simulink subsystem "ALU_64bit_v2_SS"  (R2022a)
settings: Solver=VariableStepAuto  StartTime=0.0  StopTime=10.0  RelTol=1e-3
libraries: hdlBasic x192
(part 1 of 3)
settings Model: Creator=viktor  LastModifiedBy=viktor

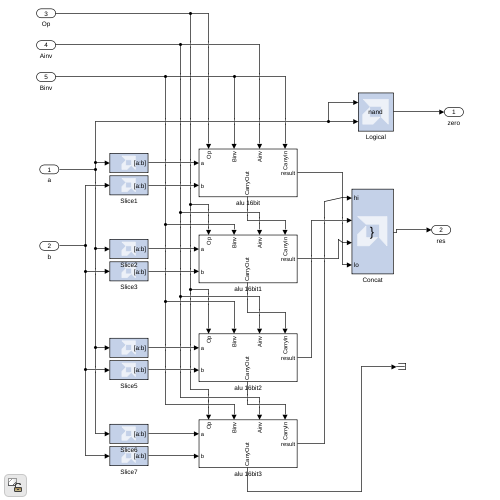
[thumbnail: Simulink's stored preview of the top-level diagram]
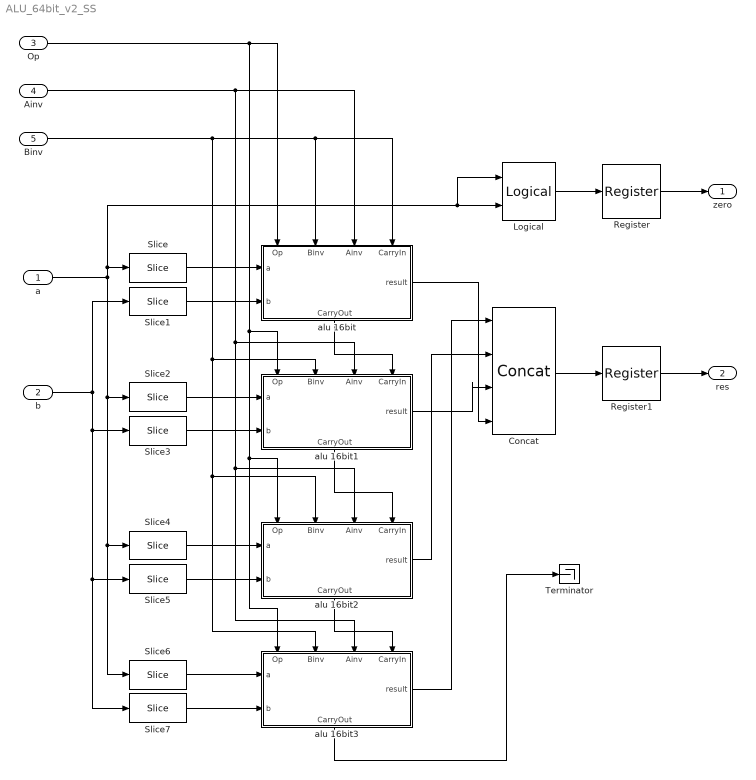
== system ALU_64bit_v2_SS ==
  a : Inport
  b : Inport  Port=2
  Op : Inport  Port=3
  Ainv : Inport  Port=4
  Binv : Inport  Port=5
  Concat : hdlBasic/Concat  num_inputs=4  XmcBlockStatus=1  maskContainerNames=group1  block_type=concat  block_config=sysgen:Concat_config
  Logical : hdlBasic/Logical  logical_function=NAND  inputs=2  en=off  latency=0  precision=User Defined  arith_type=Boolean  n_bits=16  bin_pt=0  align_bp=on  overflow=[]  quantization=[]  XmcBlockStatus=1  maskContainerNames=tabcontainer1  block_type=logical  block_config=sysgen:Logical_config
  Register : hdlBasic/Register  init=0  rst=off  en=off  XmcBlockStatus=1  maskContainerNames=tabcontainer1  block_type=register  block_config=sysgen:Register_config
  Register1 : hdlBasic/Register  init=0  rst=off  en=off  XmcBlockStatus=1  maskContainerNames=tabcontainer1  block_type=register  block_config=sysgen:Register_config
  Slice : hdlBasic/Slice  nbits=1  boolean_output=off  mode=Two Bit Locations  bit1=15  base1=LSB of Input  bit0=0  base0=LSB of Input  XmcBlockStatus=1  maskContainerNames=group1  block_type=slice  block_config=sysgen:Slice_config
  Slice1 : hdlBasic/Slice  nbits=1  boolean_output=off  mode=Two Bit Locations  bit1=15  base1=LSB of Input  bit0=0  base0=LSB of Input  XmcBlockStatus=1  maskContainerNames=group1  block_type=slice  block_config=sysgen:Slice_config
  Slice2 : hdlBasic/Slice  nbits=1  boolean_output=off  mode=Two Bit Locations  bit1=31  base1=LSB of Input  bit0=16  base0=LSB of Input  XmcBlockStatus=1  maskContainerNames=group1  block_type=slice  block_config=sysgen:Slice_config
  Slice3 : hdlBasic/Slice  nbits=1  boolean_output=off  mode=Two Bit Locations  bit1=31  base1=LSB of Input  bit0=16  base0=LSB of Input  XmcBlockStatus=1  maskContainerNames=group1  block_type=slice  block_config=sysgen:Slice_config
  Slice4 : hdlBasic/Slice  nbits=1  boolean_output=off  mode=Two Bit Locations  bit1=47  base1=LSB of Input  bit0=32  base0=LSB of Input  XmcBlockStatus=1  maskContainerNames=group1  block_type=slice  block_config=sysgen:Slice_config
  Slice5 : hdlBasic/Slice  nbits=1  boolean_output=off  mode=Two Bit Locations  bit1=47  base1=LSB of Input  bit0=32  base0=LSB of Input  XmcBlockStatus=1  maskContainerNames=group1  block_type=slice  block_config=sysgen:Slice_config
  Slice6 : hdlBasic/Slice  nbits=1  boolean_output=off  mode=Two Bit Locations  bit1=63  base1=LSB of Input  bit0=48  base0=LSB of Input  XmcBlockStatus=1  maskContainerNames=group1  block_type=slice  block_config=sysgen:Slice_config
  Slice7 : hdlBasic/Slice  nbits=1  boolean_output=off  mode=Two Bit Locations  bit1=63  base1=LSB of Input  bit0=48  base0=LSB of Input  XmcBlockStatus=1  maskContainerNames=group1  block_type=slice  block_config=sysgen:Slice_config
  Terminator : Terminator
  alu 16bit : Subsystem
      settings: PortSchema="{\"entries\":[{\"content\":{\"sides\":[{\"content\":{\"connectorIds\":[\"In1\",\"In2\"]},\"type\":\"ConnectorPlacement.EquallySpacedRectSide\",\"uuid\":\"2d8c2f3b-1550-46fa-bff2-1c6af3b5a107\"},{\"content\":{\"connectorIds\":[\"Out1\"],\"side\":\"RIGHT\"},\"type\":\"ConnectorPlacement.EquallySpacedRectSide\",\"uuid\":\"4b8f41aa-218a-4e29-bd3a-77a8547f4b37\"},{\"content\":{\"connectorIds\":[\"In3\",\"In4\",\"In5\",\"In6\"],\"side\":\"TOP\"},\"type\":\"ConnectorPlacement.EquallySpacedRectSide\",\"uuid\":\"e119eb8d-dd79-436a-880b-8e6ed91d7b6a\"},{\"content\":{\"connectorIds\":[\"Out2\"],\"side\":\"BOTTOM\"},\"type\":\"ConnectorPlacement.EquallySpacedRectSide\",\"uuid\":\"719cfc2d-1a88-4ba6-b6fd-9ae312fb718e\"}]},\"type\":\"ConnectorPlacement.EquallySpacedConnector\",\"uuid\":\"6756e4eb-c638-4708-925d-61f35342c635\"}],\"packageUris\":[\"http://schema.mathworks.com/mf0/Connector/R2020b\"],\"version\":\"1.0\"}"
  alu 16bit1 : Subsystem
      settings: PortSchema="{\"entries\":[{\"content\":{\"sides\":[{\"content\":{\"connectorIds\":[\"In1\",\"In2\"]},\"type\":\"ConnectorPlacement.EquallySpacedRectSide\",\"uuid\":\"2d8c2f3b-1550-46fa-bff2-1c6af3b5a107\"},{\"content\":{\"connectorIds\":[\"Out1\"],\"side\":\"RIGHT\"},\"type\":\"ConnectorPlacement.EquallySpacedRectSide\",\"uuid\":\"4b8f41aa-218a-4e29-bd3a-77a8547f4b37\"},{\"content\":{\"connectorIds\":[\"In3\",\"In4\",\"In5\",\"In6\"],\"side\":\"TOP\"},\"type\":\"ConnectorPlacement.EquallySpacedRectSide\",\"uuid\":\"e119eb8d-dd79-436a-880b-8e6ed91d7b6a\"},{\"content\":{\"connectorIds\":[\"Out2\"],\"side\":\"BOTTOM\"},\"type\":\"ConnectorPlacement.EquallySpacedRectSide\",\"uuid\":\"719cfc2d-1a88-4ba6-b6fd-9ae312fb718e\"}]},\"type\":\"ConnectorPlacement.EquallySpacedConnector\",\"uuid\":\"6756e4eb-c638-4708-925d-61f35342c635\"}],\"packageUris\":[\"http://schema.mathworks.com/mf0/Connector/R2020b\"],\"version\":\"1.0\"}"
  alu 16bit2 : Subsystem
      settings: PortSchema="{\"entries\":[{\"content\":{\"sides\":[{\"content\":{\"connectorIds\":[\"In1\",\"In2\"]},\"type\":\"ConnectorPlacement.EquallySpacedRectSide\",\"uuid\":\"2d8c2f3b-1550-46fa-bff2-1c6af3b5a107\"},{\"content\":{\"connectorIds\":[\"Out1\"],\"side\":\"RIGHT\"},\"type\":\"ConnectorPlacement.EquallySpacedRectSide\",\"uuid\":\"4b8f41aa-218a-4e29-bd3a-77a8547f4b37\"},{\"content\":{\"connectorIds\":[\"In3\",\"In4\",\"In5\",\"In6\"],\"side\":\"TOP\"},\"type\":\"ConnectorPlacement.EquallySpacedRectSide\",\"uuid\":\"e119eb8d-dd79-436a-880b-8e6ed91d7b6a\"},{\"content\":{\"connectorIds\":[\"Out2\"],\"side\":\"BOTTOM\"},\"type\":\"ConnectorPlacement.EquallySpacedRectSide\",\"uuid\":\"719cfc2d-1a88-4ba6-b6fd-9ae312fb718e\"}]},\"type\":\"ConnectorPlacement.EquallySpacedConnector\",\"uuid\":\"6756e4eb-c638-4708-925d-61f35342c635\"}],\"packageUris\":[\"http://schema.mathworks.com/mf0/Connector/R2020b\"],\"version\":\"1.0\"}"
  alu 16bit3 : Subsystem
      settings: PortSchema="{\"entries\":[{\"content\":{\"sides\":[{\"content\":{\"connectorIds\":[\"In1\",\"In2\"]},\"type\":\"ConnectorPlacement.EquallySpacedRectSide\",\"uuid\":\"2d8c2f3b-1550-46fa-bff2-1c6af3b5a107\"},{\"content\":{\"connectorIds\":[\"Out1\"],\"side\":\"RIGHT\"},\"type\":\"ConnectorPlacement.EquallySpacedRectSide\",\"uuid\":\"4b8f41aa-218a-4e29-bd3a-77a8547f4b37\"},{\"content\":{\"connectorIds\":[\"In3\",\"In4\",\"In5\",\"In6\"],\"side\":\"TOP\"},\"type\":\"ConnectorPlacement.EquallySpacedRectSide\",\"uuid\":\"e119eb8d-dd79-436a-880b-8e6ed91d7b6a\"},{\"content\":{\"connectorIds\":[\"Out2\"],\"side\":\"BOTTOM\"},\"type\":\"ConnectorPlacement.EquallySpacedRectSide\",\"uuid\":\"719cfc2d-1a88-4ba6-b6fd-9ae312fb718e\"}]},\"type\":\"ConnectorPlacement.EquallySpacedConnector\",\"uuid\":\"6756e4eb-c638-4708-925d-61f35342c635\"}],\"packageUris\":[\"http://schema.mathworks.com/mf0/Connector/R2020b\"],\"version\":\"1.0\"}"
  zero : Outport
  res : Outport  Port=2
  wires:
  Slice4/1 -> alu 16bit2/1(a)
  alu 16bit1/2(CarryOut) -> alu 16bit2/6(CarryIn)
  Slice1/1 -> alu 16bit/2(b)
  Slice6/1 -> alu 16bit3/1(a)
  alu 16bit3/2(CarryOut) -> Terminator/1
  Slice/1 -> alu 16bit/1(a)
  alu 16bit2/1(result) -> Concat/2
  Slice5/1 -> alu 16bit2/2(b)
  b/1 -> Slice1/1, Slice3/1, Slice5/1, Slice7/1
  Slice7/1 -> alu 16bit3/2(b)
  Slice2/1 -> alu 16bit1/1(a)
  alu 16bit2/2(CarryOut) -> alu 16bit3/6(CarryIn)
  Ainv/1 -> alu 16bit/5(Ainv), alu 16bit1/5(Ainv), alu 16bit2/5(Ainv), alu 16bit3/5(Ainv)
  a/1 -> Logical/1, Logical/2, Slice/1, Slice2/1, Slice4/1, Slice6/1
  alu 16bit1/1(result) -> Concat/3
  Slice3/1 -> alu 16bit1/2(b)
  alu 16bit/2(CarryOut) -> alu 16bit1/6(CarryIn)
  Op/1 -> alu 16bit/3(Op), alu 16bit1/3(Op), alu 16bit2/3(Op), alu 16bit3/3(Op)
  Logical/1 -> Register/1
  Binv/1 -> alu 16bit/6(CarryIn), alu 16bit/4(Binv), alu 16bit1/4(Binv), alu 16bit2/4(Binv), alu 16bit3/4(Binv)
  alu 16bit/1(result) -> Concat/4
  alu 16bit3/1(result) -> Concat/1
  Register/1 -> zero/1
  Concat/1 -> Register1/1
  Register1/1 -> res/1

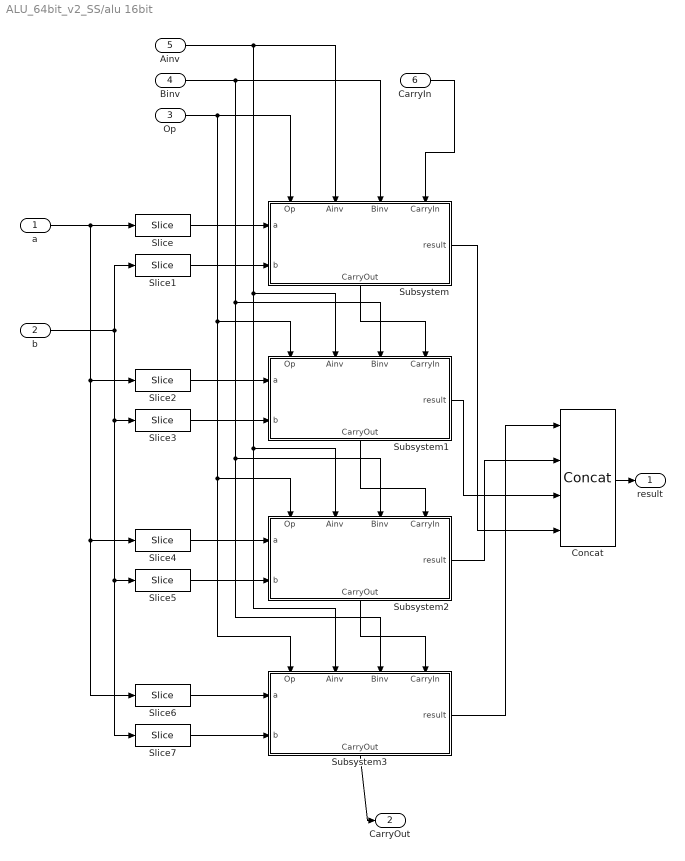
== system ALU_64bit_v2_SS/alu 16bit ==
  a : Inport
  b : Inport  Port=2
  Op : Inport  Port=3
  Binv : Inport  Port=4
  Ainv : Inport  Port=5
  CarryIn : Inport  Port=6
  Concat : hdlBasic/Concat  num_inputs=4  XmcBlockStatus=1  maskContainerNames=group1  block_type=concat  block_config=sysgen:Concat_config
  Slice : hdlBasic/Slice  nbits=1  boolean_output=off  mode=Two Bit Locations  bit1=3  base1=LSB of Input  bit0=0  base0=LSB of Input  XmcBlockStatus=1  maskContainerNames=group1  block_type=slice  block_config=sysgen:Slice_config
  Slice1 : hdlBasic/Slice  nbits=1  boolean_output=off  mode=Two Bit Locations  bit1=3  base1=LSB of Input  bit0=0  base0=LSB of Input  XmcBlockStatus=1  maskContainerNames=group1  block_type=slice  block_config=sysgen:Slice_config
  Slice2 : hdlBasic/Slice  nbits=1  boolean_output=off  mode=Two Bit Locations  bit1=7  base1=LSB of Input  bit0=4  base0=LSB of Input  XmcBlockStatus=1  maskContainerNames=group1  block_type=slice  block_config=sysgen:Slice_config
  Slice3 : hdlBasic/Slice  nbits=1  boolean_output=off  mode=Two Bit Locations  bit1=7  base1=LSB of Input  bit0=4  base0=LSB of Input  XmcBlockStatus=1  maskContainerNames=group1  block_type=slice  block_config=sysgen:Slice_config
  Slice4 : hdlBasic/Slice  nbits=1  boolean_output=off  mode=Two Bit Locations  bit1=11  base1=LSB of Input  bit0=8  base0=LSB of Input  XmcBlockStatus=1  maskContainerNames=group1  block_type=slice  block_config=sysgen:Slice_config
  Slice5 : hdlBasic/Slice  nbits=1  boolean_output=off  mode=Two Bit Locations  bit1=11  base1=LSB of Input  bit0=8  base0=LSB of Input  XmcBlockStatus=1  maskContainerNames=group1  block_type=slice  block_config=sysgen:Slice_config
  Slice6 : hdlBasic/Slice  nbits=1  boolean_output=off  mode=Two Bit Locations  bit1=15  base1=LSB of Input  bit0=12  base0=LSB of Input  XmcBlockStatus=1  maskContainerNames=group1  block_type=slice  block_config=sysgen:Slice_config
  Slice7 : hdlBasic/Slice  nbits=1  boolean_output=off  mode=Two Bit Locations  bit1=15  base1=LSB of Input  bit0=12  base0=LSB of Input  XmcBlockStatus=1  maskContainerNames=group1  block_type=slice  block_config=sysgen:Slice_config
  Subsystem : Subsystem
      settings: PortSchema="{\"entries\":[{\"content\":{\"sides\":[{\"content\":{\"connectorIds\":[\"In1\",\"In2\"]},\"type\":\"ConnectorPlacement.EquallySpacedRectSide\",\"uuid\":\"2d8c2f3b-1550-46fa-bff2-1c6af3b5a107\"},{\"content\":{\"connectorIds\":[\"Out1\"],\"side\":\"RIGHT\"},\"type\":\"ConnectorPlacement.EquallySpacedRectSide\",\"uuid\":\"4b8f41aa-218a-4e29-bd3a-77a8547f4b37\"},{\"content\":{\"connectorIds\":[\"In3\",\"In4\",\"In5\",\"In6\"],\"side\":\"TOP\"},\"type\":\"ConnectorPlacement.EquallySpacedRectSide\",\"uuid\":\"e119eb8d-dd79-436a-880b-8e6ed91d7b6a\"},{\"content\":{\"connectorIds\":[\"Out2\"],\"side\":\"BOTTOM\"},\"type\":\"ConnectorPlacement.EquallySpacedRectSide\",\"uuid\":\"1d45baa7-6d44-42d8-8289-fca13db264c9\"}]},\"type\":\"ConnectorPlacement.EquallySpacedConnector\",\"uuid\":\"6756e4eb-c638-4708-925d-61f35342c635\"}],\"packageUris\":[\"http://schema.mathworks.com/mf0/Connector/R2020b\"],\"version\":\"1.0\"}"
  Subsystem1 : Subsystem
      settings: PortSchema="{\"entries\":[{\"content\":{\"sides\":[{\"content\":{\"connectorIds\":[\"In1\",\"In2\"]},\"type\":\"ConnectorPlacement.EquallySpacedRectSide\",\"uuid\":\"2d8c2f3b-1550-46fa-bff2-1c6af3b5a107\"},{\"content\":{\"connectorIds\":[\"Out1\"],\"side\":\"RIGHT\"},\"type\":\"ConnectorPlacement.EquallySpacedRectSide\",\"uuid\":\"4b8f41aa-218a-4e29-bd3a-77a8547f4b37\"},{\"content\":{\"connectorIds\":[\"In3\",\"In4\",\"In5\",\"In6\"],\"side\":\"TOP\"},\"type\":\"ConnectorPlacement.EquallySpacedRectSide\",\"uuid\":\"e119eb8d-dd79-436a-880b-8e6ed91d7b6a\"},{\"content\":{\"connectorIds\":[\"Out2\"],\"side\":\"BOTTOM\"},\"type\":\"ConnectorPlacement.EquallySpacedRectSide\",\"uuid\":\"1d45baa7-6d44-42d8-8289-fca13db264c9\"}]},\"type\":\"ConnectorPlacement.EquallySpacedConnector\",\"uuid\":\"6756e4eb-c638-4708-925d-61f35342c635\"}],\"packageUris\":[\"http://schema.mathworks.com/mf0/Connector/R2020b\"],\"version\":\"1.0\"}"
  Subsystem2 : Subsystem
      settings: PortSchema="{\"entries\":[{\"content\":{\"sides\":[{\"content\":{\"connectorIds\":[\"In1\",\"In2\"]},\"type\":\"ConnectorPlacement.EquallySpacedRectSide\",\"uuid\":\"2d8c2f3b-1550-46fa-bff2-1c6af3b5a107\"},{\"content\":{\"connectorIds\":[\"Out1\"],\"side\":\"RIGHT\"},\"type\":\"ConnectorPlacement.EquallySpacedRectSide\",\"uuid\":\"4b8f41aa-218a-4e29-bd3a-77a8547f4b37\"},{\"content\":{\"connectorIds\":[\"In3\",\"In4\",\"In5\",\"In6\"],\"side\":\"TOP\"},\"type\":\"ConnectorPlacement.EquallySpacedRectSide\",\"uuid\":\"e119eb8d-dd79-436a-880b-8e6ed91d7b6a\"},{\"content\":{\"connectorIds\":[\"Out2\"],\"side\":\"BOTTOM\"},\"type\":\"ConnectorPlacement.EquallySpacedRectSide\",\"uuid\":\"1d45baa7-6d44-42d8-8289-fca13db264c9\"}]},\"type\":\"ConnectorPlacement.EquallySpacedConnector\",\"uuid\":\"6756e4eb-c638-4708-925d-61f35342c635\"}],\"packageUris\":[\"http://schema.mathworks.com/mf0/Connector/R2020b\"],\"version\":\"1.0\"}"
  Subsystem3 : Subsystem
      settings: PortSchema="{\"entries\":[{\"content\":{\"sides\":[{\"content\":{\"connectorIds\":[\"In1\",\"In2\"]},\"type\":\"ConnectorPlacement.EquallySpacedRectSide\",\"uuid\":\"2d8c2f3b-1550-46fa-bff2-1c6af3b5a107\"},{\"content\":{\"connectorIds\":[\"Out1\"],\"side\":\"RIGHT\"},\"type\":\"ConnectorPlacement.EquallySpacedRectSide\",\"uuid\":\"4b8f41aa-218a-4e29-bd3a-77a8547f4b37\"},{\"content\":{\"connectorIds\":[\"In3\",\"In4\",\"In5\",\"In6\"],\"side\":\"TOP\"},\"type\":\"ConnectorPlacement.EquallySpacedRectSide\",\"uuid\":\"e119eb8d-dd79-436a-880b-8e6ed91d7b6a\"},{\"content\":{\"connectorIds\":[\"Out2\"],\"side\":\"BOTTOM\"},\"type\":\"ConnectorPlacement.EquallySpacedRectSide\",\"uuid\":\"1d45baa7-6d44-42d8-8289-fca13db264c9\"}]},\"type\":\"ConnectorPlacement.EquallySpacedConnector\",\"uuid\":\"6756e4eb-c638-4708-925d-61f35342c635\"}],\"packageUris\":[\"http://schema.mathworks.com/mf0/Connector/R2020b\"],\"version\":\"1.0\"}"
  result : Outport
  CarryOut : Outport  Port=2
  wires:
  Slice/1 -> Subsystem/1(a)
  Slice2/1 -> Subsystem1/1(a)
  Subsystem/1(result) -> Concat/4
  Subsystem2/1(result) -> Concat/2
  a/1 -> Slice/1, Slice2/1, Slice4/1, Slice6/1
  b/1 -> Slice1/1, Slice3/1, Slice5/1, Slice7/1
  Concat/1 -> result/1
  Binv/1 -> Subsystem/5(Binv), Subsystem1/5(Binv), Subsystem2/5(Binv), Subsystem3/5(Binv)
  Slice7/1 -> Subsystem3/2(b)
  Subsystem3/1(result) -> Concat/1
  Subsystem3/2(CarryOut) -> CarryOut/1
  Ainv/1 -> Subsystem/4(Ainv), Subsystem1/4(Ainv), Subsystem2/4(Ainv), Subsystem3/4(Ainv)
  Op/1 -> Subsystem/3(Op), Subsystem1/3(Op), Subsystem2/3(Op), Subsystem3/3(Op)
  CarryIn/1 -> Subsystem/6(CarryIn)
  Slice5/1 -> Subsystem2/2(b)
  Slice6/1 -> Subsystem3/1(a)
  Subsystem/2(CarryOut) -> Subsystem1/6(CarryIn)
  Subsystem2/2(CarryOut) -> Subsystem3/6(CarryIn)
  Slice1/1 -> Subsystem/2(b)
  Subsystem1/2(CarryOut) -> Subsystem2/6(CarryIn)
  Subsystem1/1(result) -> Concat/3
  Slice3/1 -> Subsystem1/2(b)
  Slice4/1 -> Subsystem2/1(a)

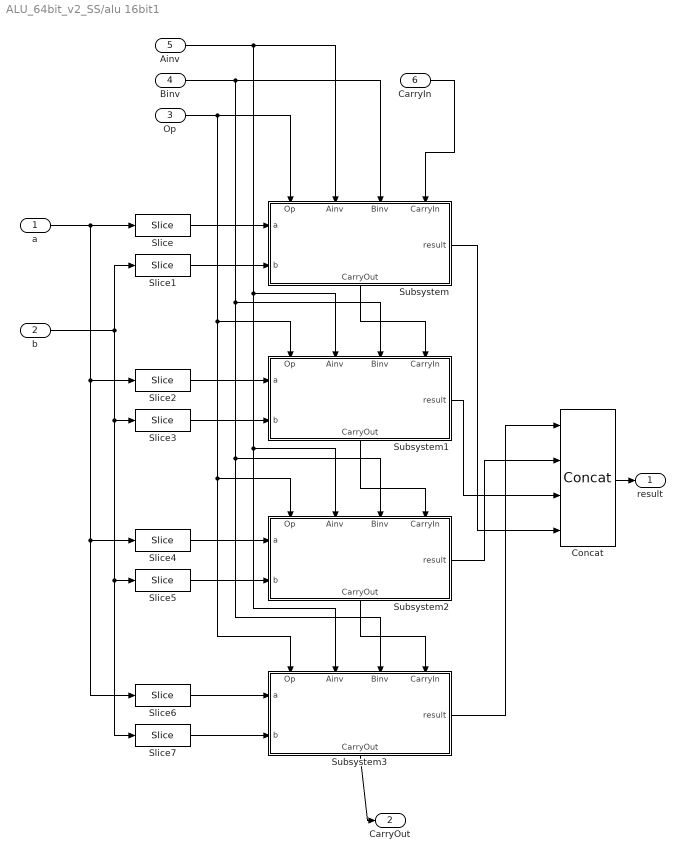
== system ALU_64bit_v2_SS/alu 16bit1 ==
  a : Inport
  b : Inport  Port=2
  Op : Inport  Port=3
  Binv : Inport  Port=4
  Ainv : Inport  Port=5
  CarryIn : Inport  Port=6
  Concat : hdlBasic/Concat  num_inputs=4  XmcBlockStatus=1  maskContainerNames=group1  block_type=concat  block_config=sysgen:Concat_config
  Slice : hdlBasic/Slice  nbits=1  boolean_output=off  mode=Two Bit Locations  bit1=3  base1=LSB of Input  bit0=0  base0=LSB of Input  XmcBlockStatus=1  maskContainerNames=group1  block_type=slice  block_config=sysgen:Slice_config
  Slice1 : hdlBasic/Slice  nbits=1  boolean_output=off  mode=Two Bit Locations  bit1=3  base1=LSB of Input  bit0=0  base0=LSB of Input  XmcBlockStatus=1  maskContainerNames=group1  block_type=slice  block_config=sysgen:Slice_config
  Slice2 : hdlBasic/Slice  nbits=1  boolean_output=off  mode=Two Bit Locations  bit1=7  base1=LSB of Input  bit0=4  base0=LSB of Input  XmcBlockStatus=1  maskContainerNames=group1  block_type=slice  block_config=sysgen:Slice_config
  Slice3 : hdlBasic/Slice  nbits=1  boolean_output=off  mode=Two Bit Locations  bit1=7  base1=LSB of Input  bit0=4  base0=LSB of Input  XmcBlockStatus=1  maskContainerNames=group1  block_type=slice  block_config=sysgen:Slice_config
  Slice4 : hdlBasic/Slice  nbits=1  boolean_output=off  mode=Two Bit Locations  bit1=11  base1=LSB of Input  bit0=8  base0=LSB of Input  XmcBlockStatus=1  maskContainerNames=group1  block_type=slice  block_config=sysgen:Slice_config
  Slice5 : hdlBasic/Slice  nbits=1  boolean_output=off  mode=Two Bit Locations  bit1=11  base1=LSB of Input  bit0=8  base0=LSB of Input  XmcBlockStatus=1  maskContainerNames=group1  block_type=slice  block_config=sysgen:Slice_config
  Slice6 : hdlBasic/Slice  nbits=1  boolean_output=off  mode=Two Bit Locations  bit1=15  base1=LSB of Input  bit0=12  base0=LSB of Input  XmcBlockStatus=1  maskContainerNames=group1  block_type=slice  block_config=sysgen:Slice_config
  Slice7 : hdlBasic/Slice  nbits=1  boolean_output=off  mode=Two Bit Locations  bit1=15  base1=LSB of Input  bit0=12  base0=LSB of Input  XmcBlockStatus=1  maskContainerNames=group1  block_type=slice  block_config=sysgen:Slice_config
  Subsystem : Subsystem
      settings: PortSchema="{\"entries\":[{\"content\":{\"sides\":[{\"content\":{\"connectorIds\":[\"In1\",\"In2\"]},\"type\":\"ConnectorPlacement.EquallySpacedRectSide\",\"uuid\":\"2d8c2f3b-1550-46fa-bff2-1c6af3b5a107\"},{\"content\":{\"connectorIds\":[\"Out1\"],\"side\":\"RIGHT\"},\"type\":\"ConnectorPlacement.EquallySpacedRectSide\",\"uuid\":\"4b8f41aa-218a-4e29-bd3a-77a8547f4b37\"},{\"content\":{\"connectorIds\":[\"In3\",\"In4\",\"In5\",\"In6\"],\"side\":\"TOP\"},\"type\":\"ConnectorPlacement.EquallySpacedRectSide\",\"uuid\":\"e119eb8d-dd79-436a-880b-8e6ed91d7b6a\"},{\"content\":{\"connectorIds\":[\"Out2\"],\"side\":\"BOTTOM\"},\"type\":\"ConnectorPlacement.EquallySpacedRectSide\",\"uuid\":\"1d45baa7-6d44-42d8-8289-fca13db264c9\"}]},\"type\":\"ConnectorPlacement.EquallySpacedConnector\",\"uuid\":\"6756e4eb-c638-4708-925d-61f35342c635\"}],\"packageUris\":[\"http://schema.mathworks.com/mf0/Connector/R2020b\"],\"version\":\"1.0\"}"
  Subsystem1 : Subsystem
      settings: PortSchema="{\"entries\":[{\"content\":{\"sides\":[{\"content\":{\"connectorIds\":[\"In1\",\"In2\"]},\"type\":\"ConnectorPlacement.EquallySpacedRectSide\",\"uuid\":\"2d8c2f3b-1550-46fa-bff2-1c6af3b5a107\"},{\"content\":{\"connectorIds\":[\"Out1\"],\"side\":\"RIGHT\"},\"type\":\"ConnectorPlacement.EquallySpacedRectSide\",\"uuid\":\"4b8f41aa-218a-4e29-bd3a-77a8547f4b37\"},{\"content\":{\"connectorIds\":[\"In3\",\"In4\",\"In5\",\"In6\"],\"side\":\"TOP\"},\"type\":\"ConnectorPlacement.EquallySpacedRectSide\",\"uuid\":\"e119eb8d-dd79-436a-880b-8e6ed91d7b6a\"},{\"content\":{\"connectorIds\":[\"Out2\"],\"side\":\"BOTTOM\"},\"type\":\"ConnectorPlacement.EquallySpacedRectSide\",\"uuid\":\"1d45baa7-6d44-42d8-8289-fca13db264c9\"}]},\"type\":\"ConnectorPlacement.EquallySpacedConnector\",\"uuid\":\"6756e4eb-c638-4708-925d-61f35342c635\"}],\"packageUris\":[\"http://schema.mathworks.com/mf0/Connector/R2020b\"],\"version\":\"1.0\"}"
  Subsystem2 : Subsystem
      settings: PortSchema="{\"entries\":[{\"content\":{\"sides\":[{\"content\":{\"connectorIds\":[\"In1\",\"In2\"]},\"type\":\"ConnectorPlacement.EquallySpacedRectSide\",\"uuid\":\"2d8c2f3b-1550-46fa-bff2-1c6af3b5a107\"},{\"content\":{\"connectorIds\":[\"Out1\"],\"side\":\"RIGHT\"},\"type\":\"ConnectorPlacement.EquallySpacedRectSide\",\"uuid\":\"4b8f41aa-218a-4e29-bd3a-77a8547f4b37\"},{\"content\":{\"connectorIds\":[\"In3\",\"In4\",\"In5\",\"In6\"],\"side\":\"TOP\"},\"type\":\"ConnectorPlacement.EquallySpacedRectSide\",\"uuid\":\"e119eb8d-dd79-436a-880b-8e6ed91d7b6a\"},{\"content\":{\"connectorIds\":[\"Out2\"],\"side\":\"BOTTOM\"},\"type\":\"ConnectorPlacement.EquallySpacedRectSide\",\"uuid\":\"1d45baa7-6d44-42d8-8289-fca13db264c9\"}]},\"type\":\"ConnectorPlacement.EquallySpacedConnector\",\"uuid\":\"6756e4eb-c638-4708-925d-61f35342c635\"}],\"packageUris\":[\"http://schema.mathworks.com/mf0/Connector/R2020b\"],\"version\":\"1.0\"}"
  Subsystem3 : Subsystem
      settings: PortSchema="{\"entries\":[{\"content\":{\"sides\":[{\"content\":{\"connectorIds\":[\"In1\",\"In2\"]},\"type\":\"ConnectorPlacement.EquallySpacedRectSide\",\"uuid\":\"2d8c2f3b-1550-46fa-bff2-1c6af3b5a107\"},{\"content\":{\"connectorIds\":[\"Out1\"],\"side\":\"RIGHT\"},\"type\":\"ConnectorPlacement.EquallySpacedRectSide\",\"uuid\":\"4b8f41aa-218a-4e29-bd3a-77a8547f4b37\"},{\"content\":{\"connectorIds\":[\"In3\",\"In4\",\"In5\",\"In6\"],\"side\":\"TOP\"},\"type\":\"ConnectorPlacement.EquallySpacedRectSide\",\"uuid\":\"e119eb8d-dd79-436a-880b-8e6ed91d7b6a\"},{\"content\":{\"connectorIds\":[\"Out2\"],\"side\":\"BOTTOM\"},\"type\":\"ConnectorPlacement.EquallySpacedRectSide\",\"uuid\":\"1d45baa7-6d44-42d8-8289-fca13db264c9\"}]},\"type\":\"ConnectorPlacement.EquallySpacedConnector\",\"uuid\":\"6756e4eb-c638-4708-925d-61f35342c635\"}],\"packageUris\":[\"http://schema.mathworks.com/mf0/Connector/R2020b\"],\"version\":\"1.0\"}"
  result : Outport
  CarryOut : Outport  Port=2
  wires:
  Slice/1 -> Subsystem/1(a)
  Slice2/1 -> Subsystem1/1(a)
  Subsystem/1(result) -> Concat/4
  Subsystem2/1(result) -> Concat/2
  a/1 -> Slice/1, Slice2/1, Slice4/1, Slice6/1
  b/1 -> Slice1/1, Slice3/1, Slice5/1, Slice7/1
  Concat/1 -> result/1
  Binv/1 -> Subsystem/5(Binv), Subsystem1/5(Binv), Subsystem2/5(Binv), Subsystem3/5(Binv)
  Slice7/1 -> Subsystem3/2(b)
  Subsystem3/1(result) -> Concat/1
  Subsystem3/2(CarryOut) -> CarryOut/1
  Ainv/1 -> Subsystem/4(Ainv), Subsystem1/4(Ainv), Subsystem2/4(Ainv), Subsystem3/4(Ainv)
  Op/1 -> Subsystem/3(Op), Subsystem1/3(Op), Subsystem2/3(Op), Subsystem3/3(Op)
  CarryIn/1 -> Subsystem/6(CarryIn)
  Slice5/1 -> Subsystem2/2(b)
  Slice6/1 -> Subsystem3/1(a)
  Subsystem/2(CarryOut) -> Subsystem1/6(CarryIn)
  Subsystem2/2(CarryOut) -> Subsystem3/6(CarryIn)
  Slice1/1 -> Subsystem/2(b)
  Subsystem1/2(CarryOut) -> Subsystem2/6(CarryIn)
  Subsystem1/1(result) -> Concat/3
  Slice3/1 -> Subsystem1/2(b)
  Slice4/1 -> Subsystem2/1(a)

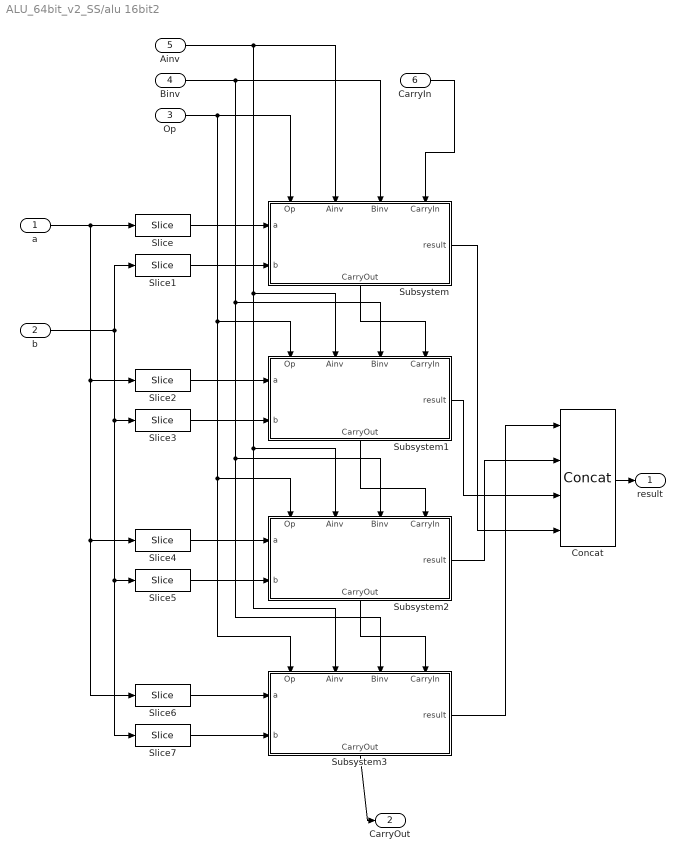
== system ALU_64bit_v2_SS/alu 16bit2 ==
  a : Inport
  b : Inport  Port=2
  Op : Inport  Port=3
  Binv : Inport  Port=4
  Ainv : Inport  Port=5
  CarryIn : Inport  Port=6
  Concat : hdlBasic/Concat  num_inputs=4  XmcBlockStatus=1  maskContainerNames=group1  block_type=concat  block_config=sysgen:Concat_config
  Slice : hdlBasic/Slice  nbits=1  boolean_output=off  mode=Two Bit Locations  bit1=3  base1=LSB of Input  bit0=0  base0=LSB of Input  XmcBlockStatus=1  maskContainerNames=group1  block_type=slice  block_config=sysgen:Slice_config
  Slice1 : hdlBasic/Slice  nbits=1  boolean_output=off  mode=Two Bit Locations  bit1=3  base1=LSB of Input  bit0=0  base0=LSB of Input  XmcBlockStatus=1  maskContainerNames=group1  block_type=slice  block_config=sysgen:Slice_config
  Slice2 : hdlBasic/Slice  nbits=1  boolean_output=off  mode=Two Bit Locations  bit1=7  base1=LSB of Input  bit0=4  base0=LSB of Input  XmcBlockStatus=1  maskContainerNames=group1  block_type=slice  block_config=sysgen:Slice_config
  Slice3 : hdlBasic/Slice  nbits=1  boolean_output=off  mode=Two Bit Locations  bit1=7  base1=LSB of Input  bit0=4  base0=LSB of Input  XmcBlockStatus=1  maskContainerNames=group1  block_type=slice  block_config=sysgen:Slice_config
  Slice4 : hdlBasic/Slice  nbits=1  boolean_output=off  mode=Two Bit Locations  bit1=11  base1=LSB of Input  bit0=8  base0=LSB of Input  XmcBlockStatus=1  maskContainerNames=group1  block_type=slice  block_config=sysgen:Slice_config
  Slice5 : hdlBasic/Slice  nbits=1  boolean_output=off  mode=Two Bit Locations  bit1=11  base1=LSB of Input  bit0=8  base0=LSB of Input  XmcBlockStatus=1  maskContainerNames=group1  block_type=slice  block_config=sysgen:Slice_config
  Slice6 : hdlBasic/Slice  nbits=1  boolean_output=off  mode=Two Bit Locations  bit1=15  base1=LSB of Input  bit0=12  base0=LSB of Input  XmcBlockStatus=1  maskContainerNames=group1  block_type=slice  block_config=sysgen:Slice_config
  Slice7 : hdlBasic/Slice  nbits=1  boolean_output=off  mode=Two Bit Locations  bit1=15  base1=LSB of Input  bit0=12  base0=LSB of Input  XmcBlockStatus=1  maskContainerNames=group1  block_type=slice  block_config=sysgen:Slice_config
  Subsystem : Subsystem
      settings: PortSchema="{\"entries\":[{\"content\":{\"sides\":[{\"content\":{\"connectorIds\":[\"In1\",\"In2\"]},\"type\":\"ConnectorPlacement.EquallySpacedRectSide\",\"uuid\":\"2d8c2f3b-1550-46fa-bff2-1c6af3b5a107\"},{\"content\":{\"connectorIds\":[\"Out1\"],\"side\":\"RIGHT\"},\"type\":\"ConnectorPlacement.EquallySpacedRectSide\",\"uuid\":\"4b8f41aa-218a-4e29-bd3a-77a8547f4b37\"},{\"content\":{\"connectorIds\":[\"In3\",\"In4\",\"In5\",\"In6\"],\"side\":\"TOP\"},\"type\":\"ConnectorPlacement.EquallySpacedRectSide\",\"uuid\":\"e119eb8d-dd79-436a-880b-8e6ed91d7b6a\"},{\"content\":{\"connectorIds\":[\"Out2\"],\"side\":\"BOTTOM\"},\"type\":\"ConnectorPlacement.EquallySpacedRectSide\",\"uuid\":\"1d45baa7-6d44-42d8-8289-fca13db264c9\"}]},\"type\":\"ConnectorPlacement.EquallySpacedConnector\",\"uuid\":\"6756e4eb-c638-4708-925d-61f35342c635\"}],\"packageUris\":[\"http://schema.mathworks.com/mf0/Connector/R2020b\"],\"version\":\"1.0\"}"
  Subsystem1 : Subsystem
      settings: PortSchema="{\"entries\":[{\"content\":{\"sides\":[{\"content\":{\"connectorIds\":[\"In1\",\"In2\"]},\"type\":\"ConnectorPlacement.EquallySpacedRectSide\",\"uuid\":\"2d8c2f3b-1550-46fa-bff2-1c6af3b5a107\"},{\"content\":{\"connectorIds\":[\"Out1\"],\"side\":\"RIGHT\"},\"type\":\"ConnectorPlacement.EquallySpacedRectSide\",\"uuid\":\"4b8f41aa-218a-4e29-bd3a-77a8547f4b37\"},{\"content\":{\"connectorIds\":[\"In3\",\"In4\",\"In5\",\"In6\"],\"side\":\"TOP\"},\"type\":\"ConnectorPlacement.EquallySpacedRectSide\",\"uuid\":\"e119eb8d-dd79-436a-880b-8e6ed91d7b6a\"},{\"content\":{\"connectorIds\":[\"Out2\"],\"side\":\"BOTTOM\"},\"type\":\"ConnectorPlacement.EquallySpacedRectSide\",\"uuid\":\"1d45baa7-6d44-42d8-8289-fca13db264c9\"}]},\"type\":\"ConnectorPlacement.EquallySpacedConnector\",\"uuid\":\"6756e4eb-c638-4708-925d-61f35342c635\"}],\"packageUris\":[\"http://schema.mathworks.com/mf0/Connector/R2020b\"],\"version\":\"1.0\"}"
  Subsystem2 : Subsystem
      settings: PortSchema="{\"entries\":[{\"content\":{\"sides\":[{\"content\":{\"connectorIds\":[\"In1\",\"In2\"]},\"type\":\"ConnectorPlacement.EquallySpacedRectSide\",\"uuid\":\"2d8c2f3b-1550-46fa-bff2-1c6af3b5a107\"},{\"content\":{\"connectorIds\":[\"Out1\"],\"side\":\"RIGHT\"},\"type\":\"ConnectorPlacement.EquallySpacedRectSide\",\"uuid\":\"4b8f41aa-218a-4e29-bd3a-77a8547f4b37\"},{\"content\":{\"connectorIds\":[\"In3\",\"In4\",\"In5\",\"In6\"],\"side\":\"TOP\"},\"type\":\"ConnectorPlacement.EquallySpacedRectSide\",\"uuid\":\"e119eb8d-dd79-436a-880b-8e6ed91d7b6a\"},{\"content\":{\"connectorIds\":[\"Out2\"],\"side\":\"BOTTOM\"},\"type\":\"ConnectorPlacement.EquallySpacedRectSide\",\"uuid\":\"1d45baa7-6d44-42d8-8289-fca13db264c9\"}]},\"type\":\"ConnectorPlacement.EquallySpacedConnector\",\"uuid\":\"6756e4eb-c638-4708-925d-61f35342c635\"}],\"packageUris\":[\"http://schema.mathworks.com/mf0/Connector/R2020b\"],\"version\":\"1.0\"}"
  Subsystem3 : Subsystem
      settings: PortSchema="{\"entries\":[{\"content\":{\"sides\":[{\"content\":{\"connectorIds\":[\"In1\",\"In2\"]},\"type\":\"ConnectorPlacement.EquallySpacedRectSide\",\"uuid\":\"2d8c2f3b-1550-46fa-bff2-1c6af3b5a107\"},{\"content\":{\"connectorIds\":[\"Out1\"],\"side\":\"RIGHT\"},\"type\":\"ConnectorPlacement.EquallySpacedRectSide\",\"uuid\":\"4b8f41aa-218a-4e29-bd3a-77a8547f4b37\"},{\"content\":{\"connectorIds\":[\"In3\",\"In4\",\"In5\",\"In6\"],\"side\":\"TOP\"},\"type\":\"ConnectorPlacement.EquallySpacedRectSide\",\"uuid\":\"e119eb8d-dd79-436a-880b-8e6ed91d7b6a\"},{\"content\":{\"connectorIds\":[\"Out2\"],\"side\":\"BOTTOM\"},\"type\":\"ConnectorPlacement.EquallySpacedRectSide\",\"uuid\":\"1d45baa7-6d44-42d8-8289-fca13db264c9\"}]},\"type\":\"ConnectorPlacement.EquallySpacedConnector\",\"uuid\":\"6756e4eb-c638-4708-925d-61f35342c635\"}],\"packageUris\":[\"http://schema.mathworks.com/mf0/Connector/R2020b\"],\"version\":\"1.0\"}"
  result : Outport
  CarryOut : Outport  Port=2
  wires:
  Slice/1 -> Subsystem/1(a)
  Slice2/1 -> Subsystem1/1(a)
  Subsystem/1(result) -> Concat/4
  Subsystem2/1(result) -> Concat/2
  a/1 -> Slice/1, Slice2/1, Slice4/1, Slice6/1
  b/1 -> Slice1/1, Slice3/1, Slice5/1, Slice7/1
  Concat/1 -> result/1
  Binv/1 -> Subsystem/5(Binv), Subsystem1/5(Binv), Subsystem2/5(Binv), Subsystem3/5(Binv)
  Slice7/1 -> Subsystem3/2(b)
  Subsystem3/1(result) -> Concat/1
  Subsystem3/2(CarryOut) -> CarryOut/1
  Ainv/1 -> Subsystem/4(Ainv), Subsystem1/4(Ainv), Subsystem2/4(Ainv), Subsystem3/4(Ainv)
  Op/1 -> Subsystem/3(Op), Subsystem1/3(Op), Subsystem2/3(Op), Subsystem3/3(Op)
  CarryIn/1 -> Subsystem/6(CarryIn)
  Slice5/1 -> Subsystem2/2(b)
  Slice6/1 -> Subsystem3/1(a)
  Subsystem/2(CarryOut) -> Subsystem1/6(CarryIn)
  Subsystem2/2(CarryOut) -> Subsystem3/6(CarryIn)
  Slice1/1 -> Subsystem/2(b)
  Subsystem1/2(CarryOut) -> Subsystem2/6(CarryIn)
  Subsystem1/1(result) -> Concat/3
  Slice3/1 -> Subsystem1/2(b)
  Slice4/1 -> Subsystem2/1(a)

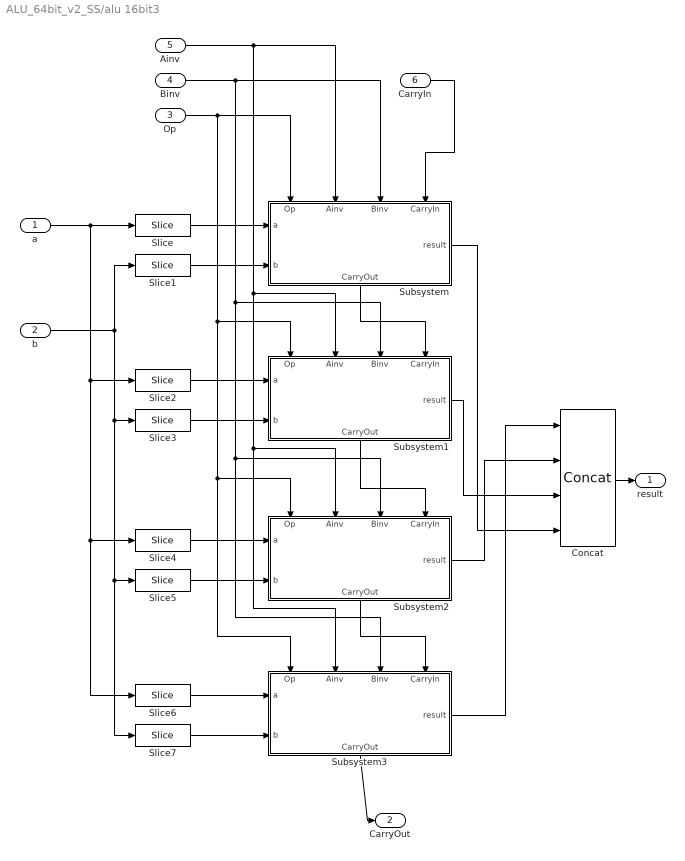
== system ALU_64bit_v2_SS/alu 16bit3 ==
  a : Inport
  b : Inport  Port=2
  Op : Inport  Port=3
  Binv : Inport  Port=4
  Ainv : Inport  Port=5
  CarryIn : Inport  Port=6
  Concat : hdlBasic/Concat  num_inputs=4  XmcBlockStatus=1  maskContainerNames=group1  block_type=concat  block_config=sysgen:Concat_config
  Slice : hdlBasic/Slice  nbits=1  boolean_output=off  mode=Two Bit Locations  bit1=3  base1=LSB of Input  bit0=0  base0=LSB of Input  XmcBlockStatus=1  maskContainerNames=group1  block_type=slice  block_config=sysgen:Slice_config
  Slice1 : hdlBasic/Slice  nbits=1  boolean_output=off  mode=Two Bit Locations  bit1=3  base1=LSB of Input  bit0=0  base0=LSB of Input  XmcBlockStatus=1  maskContainerNames=group1  block_type=slice  block_config=sysgen:Slice_config
  Slice2 : hdlBasic/Slice  nbits=1  boolean_output=off  mode=Two Bit Locations  bit1=7  base1=LSB of Input  bit0=4  base0=LSB of Input  XmcBlockStatus=1  maskContainerNames=group1  block_type=slice  block_config=sysgen:Slice_config
  Slice3 : hdlBasic/Slice  nbits=1  boolean_output=off  mode=Two Bit Locations  bit1=7  base1=LSB of Input  bit0=4  base0=LSB of Input  XmcBlockStatus=1  maskContainerNames=group1  block_type=slice  block_config=sysgen:Slice_config
  Slice4 : hdlBasic/Slice  nbits=1  boolean_output=off  mode=Two Bit Locations  bit1=11  base1=LSB of Input  bit0=8  base0=LSB of Input  XmcBlockStatus=1  maskContainerNames=group1  block_type=slice  block_config=sysgen:Slice_config
  Slice5 : hdlBasic/Slice  nbits=1  boolean_output=off  mode=Two Bit Locations  bit1=11  base1=LSB of Input  bit0=8  base0=LSB of Input  XmcBlockStatus=1  maskContainerNames=group1  block_type=slice  block_config=sysgen:Slice_config
  Slice6 : hdlBasic/Slice  nbits=1  boolean_output=off  mode=Two Bit Locations  bit1=15  base1=LSB of Input  bit0=12  base0=LSB of Input  XmcBlockStatus=1  maskContainerNames=group1  block_type=slice  block_config=sysgen:Slice_config
  Slice7 : hdlBasic/Slice  nbits=1  boolean_output=off  mode=Two Bit Locations  bit1=15  base1=LSB of Input  bit0=12  base0=LSB of Input  XmcBlockStatus=1  maskContainerNames=group1  block_type=slice  block_config=sysgen:Slice_config
  Subsystem : Subsystem
      settings: PortSchema="{\"entries\":[{\"content\":{\"sides\":[{\"content\":{\"connectorIds\":[\"In1\",\"In2\"]},\"type\":\"ConnectorPlacement.EquallySpacedRectSide\",\"uuid\":\"2d8c2f3b-1550-46fa-bff2-1c6af3b5a107\"},{\"content\":{\"connectorIds\":[\"Out1\"],\"side\":\"RIGHT\"},\"type\":\"ConnectorPlacement.EquallySpacedRectSide\",\"uuid\":\"4b8f41aa-218a-4e29-bd3a-77a8547f4b37\"},{\"content\":{\"connectorIds\":[\"In3\",\"In4\",\"In5\",\"In6\"],\"side\":\"TOP\"},\"type\":\"ConnectorPlacement.EquallySpacedRectSide\",\"uuid\":\"e119eb8d-dd79-436a-880b-8e6ed91d7b6a\"},{\"content\":{\"connectorIds\":[\"Out2\"],\"side\":\"BOTTOM\"},\"type\":\"ConnectorPlacement.EquallySpacedRectSide\",\"uuid\":\"1d45baa7-6d44-42d8-8289-fca13db264c9\"}]},\"type\":\"ConnectorPlacement.EquallySpacedConnector\",\"uuid\":\"6756e4eb-c638-4708-925d-61f35342c635\"}],\"packageUris\":[\"http://schema.mathworks.com/mf0/Connector/R2020b\"],\"version\":\"1.0\"}"
  Subsystem1 : Subsystem
      settings: PortSchema="{\"entries\":[{\"content\":{\"sides\":[{\"content\":{\"connectorIds\":[\"In1\",\"In2\"]},\"type\":\"ConnectorPlacement.EquallySpacedRectSide\",\"uuid\":\"2d8c2f3b-1550-46fa-bff2-1c6af3b5a107\"},{\"content\":{\"connectorIds\":[\"Out1\"],\"side\":\"RIGHT\"},\"type\":\"ConnectorPlacement.EquallySpacedRectSide\",\"uuid\":\"4b8f41aa-218a-4e29-bd3a-77a8547f4b37\"},{\"content\":{\"connectorIds\":[\"In3\",\"In4\",\"In5\",\"In6\"],\"side\":\"TOP\"},\"type\":\"ConnectorPlacement.EquallySpacedRectSide\",\"uuid\":\"e119eb8d-dd79-436a-880b-8e6ed91d7b6a\"},{\"content\":{\"connectorIds\":[\"Out2\"],\"side\":\"BOTTOM\"},\"type\":\"ConnectorPlacement.EquallySpacedRectSide\",\"uuid\":\"1d45baa7-6d44-42d8-8289-fca13db264c9\"}]},\"type\":\"ConnectorPlacement.EquallySpacedConnector\",\"uuid\":\"6756e4eb-c638-4708-925d-61f35342c635\"}],\"packageUris\":[\"http://schema.mathworks.com/mf0/Connector/R2020b\"],\"version\":\"1.0\"}"
  Subsystem2 : Subsystem
      settings: PortSchema="{\"entries\":[{\"content\":{\"sides\":[{\"content\":{\"connectorIds\":[\"In1\",\"In2\"]},\"type\":\"ConnectorPlacement.EquallySpacedRectSide\",\"uuid\":\"2d8c2f3b-1550-46fa-bff2-1c6af3b5a107\"},{\"content\":{\"connectorIds\":[\"Out1\"],\"side\":\"RIGHT\"},\"type\":\"ConnectorPlacement.EquallySpacedRectSide\",\"uuid\":\"4b8f41aa-218a-4e29-bd3a-77a8547f4b37\"},{\"content\":{\"connectorIds\":[\"In3\",\"In4\",\"In5\",\"In6\"],\"side\":\"TOP\"},\"type\":\"ConnectorPlacement.EquallySpacedRectSide\",\"uuid\":\"e119eb8d-dd79-436a-880b-8e6ed91d7b6a\"},{\"content\":{\"connectorIds\":[\"Out2\"],\"side\":\"BOTTOM\"},\"type\":\"ConnectorPlacement.EquallySpacedRectSide\",\"uuid\":\"1d45baa7-6d44-42d8-8289-fca13db264c9\"}]},\"type\":\"ConnectorPlacement.EquallySpacedConnector\",\"uuid\":\"6756e4eb-c638-4708-925d-61f35342c635\"}],\"packageUris\":[\"http://schema.mathworks.com/mf0/Connector/R2020b\"],\"version\":\"1.0\"}"
  Subsystem3 : Subsystem
      settings: PortSchema="{\"entries\":[{\"content\":{\"sides\":[{\"content\":{\"connectorIds\":[\"In1\",\"In2\"]},\"type\":\"ConnectorPlacement.EquallySpacedRectSide\",\"uuid\":\"2d8c2f3b-1550-46fa-bff2-1c6af3b5a107\"},{\"content\":{\"connectorIds\":[\"Out1\"],\"side\":\"RIGHT\"},\"type\":\"ConnectorPlacement.EquallySpacedRectSide\",\"uuid\":\"4b8f41aa-218a-4e29-bd3a-77a8547f4b37\"},{\"content\":{\"connectorIds\":[\"In3\",\"In4\",\"In5\",\"In6\"],\"side\":\"TOP\"},\"type\":\"ConnectorPlacement.EquallySpacedRectSide\",\"uuid\":\"e119eb8d-dd79-436a-880b-8e6ed91d7b6a\"},{\"content\":{\"connectorIds\":[\"Out2\"],\"side\":\"BOTTOM\"},\"type\":\"ConnectorPlacement.EquallySpacedRectSide\",\"uuid\":\"1d45baa7-6d44-42d8-8289-fca13db264c9\"}]},\"type\":\"ConnectorPlacement.EquallySpacedConnector\",\"uuid\":\"6756e4eb-c638-4708-925d-61f35342c635\"}],\"packageUris\":[\"http://schema.mathworks.com/mf0/Connector/R2020b\"],\"version\":\"1.0\"}"
  result : Outport
  CarryOut : Outport  Port=2
  wires:
  Slice/1 -> Subsystem/1(a)
  Slice2/1 -> Subsystem1/1(a)
  Subsystem/1(result) -> Concat/4
  Subsystem2/1(result) -> Concat/2
  a/1 -> Slice/1, Slice2/1, Slice4/1, Slice6/1
  b/1 -> Slice1/1, Slice3/1, Slice5/1, Slice7/1
  Concat/1 -> result/1
  Binv/1 -> Subsystem/5(Binv), Subsystem1/5(Binv), Subsystem2/5(Binv), Subsystem3/5(Binv)
  Slice7/1 -> Subsystem3/2(b)
  Subsystem3/1(result) -> Concat/1
  Subsystem3/2(CarryOut) -> CarryOut/1
  Ainv/1 -> Subsystem/4(Ainv), Subsystem1/4(Ainv), Subsystem2/4(Ainv), Subsystem3/4(Ainv)
  Op/1 -> Subsystem/3(Op), Subsystem1/3(Op), Subsystem2/3(Op), Subsystem3/3(Op)
  CarryIn/1 -> Subsystem/6(CarryIn)
  Slice5/1 -> Subsystem2/2(b)
  Slice6/1 -> Subsystem3/1(a)
  Subsystem/2(CarryOut) -> Subsystem1/6(CarryIn)
  Subsystem2/2(CarryOut) -> Subsystem3/6(CarryIn)
  Slice1/1 -> Subsystem/2(b)
  Subsystem1/2(CarryOut) -> Subsystem2/6(CarryIn)
  Subsystem1/1(result) -> Concat/3
  Slice3/1 -> Subsystem1/2(b)
  Slice4/1 -> Subsystem2/1(a)

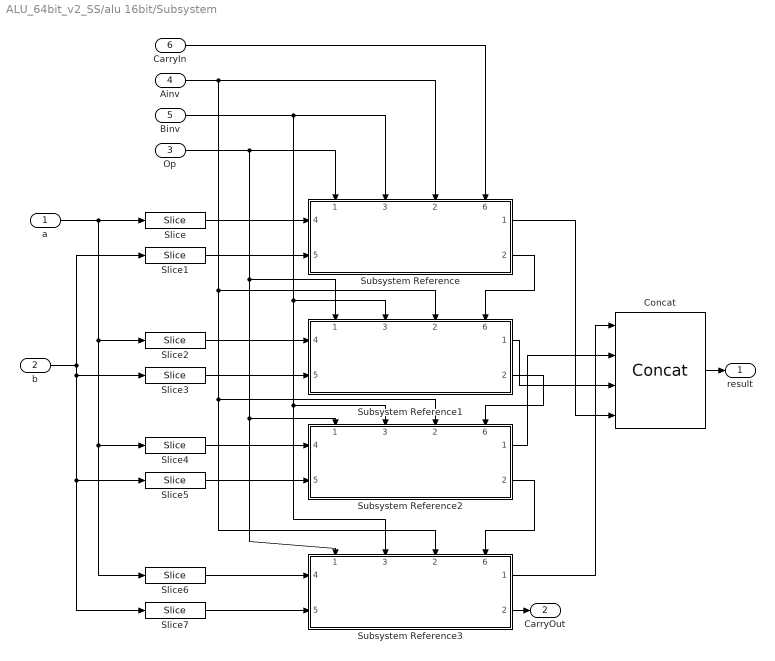
== system ALU_64bit_v2_SS/alu 16bit/Subsystem ==
  a : Inport
  b : Inport  Port=2
  Op : Inport  Port=3
  Ainv : Inport  Port=4
  Binv : Inport  Port=5
  CarryIn : Inport  Port=6
  Concat : hdlBasic/Concat  num_inputs=4  XmcBlockStatus=1  maskContainerNames=group1  block_type=concat  block_config=sysgen:Concat_config
  Slice : hdlBasic/Slice  nbits=1  boolean_output=off  mode=Upper Bit Location + Width  bit1=0  base1=LSB of Input  bit0=0  base0=LSB of Input  XmcBlockStatus=1  maskContainerNames=group1  block_type=slice  block_config=sysgen:Slice_config
  Slice1 : hdlBasic/Slice  nbits=1  boolean_output=off  mode=Upper Bit Location + Width  bit1=0  base1=LSB of Input  bit0=0  base0=LSB of Input  XmcBlockStatus=1  maskContainerNames=group1  block_type=slice  block_config=sysgen:Slice_config
  Slice2 : hdlBasic/Slice  nbits=1  boolean_output=off  mode=Upper Bit Location + Width  bit1=1  base1=LSB of Input  bit0=0  base0=LSB of Input  XmcBlockStatus=1  maskContainerNames=group1  block_type=slice  block_config=sysgen:Slice_config
  Slice3 : hdlBasic/Slice  nbits=1  boolean_output=off  mode=Upper Bit Location + Width  bit1=1  base1=LSB of Input  bit0=0  base0=LSB of Input  XmcBlockStatus=1  maskContainerNames=group1  block_type=slice  block_config=sysgen:Slice_config
  Slice4 : hdlBasic/Slice  nbits=1  boolean_output=off  mode=Upper Bit Location + Width  bit1=2  base1=LSB of Input  bit0=0  base0=LSB of Input  XmcBlockStatus=1  maskContainerNames=group1  block_type=slice  block_config=sysgen:Slice_config
  Slice5 : hdlBasic/Slice  nbits=1  boolean_output=off  mode=Upper Bit Location + Width  bit1=2  base1=LSB of Input  bit0=0  base0=LSB of Input  XmcBlockStatus=1  maskContainerNames=group1  block_type=slice  block_config=sysgen:Slice_config
  Slice6 : hdlBasic/Slice  nbits=1  boolean_output=off  mode=Upper Bit Location + Width  bit1=3  base1=LSB of Input  bit0=0  base0=LSB of Input  XmcBlockStatus=1  maskContainerNames=group1  block_type=slice  block_config=sysgen:Slice_config
  Slice7 : hdlBasic/Slice  nbits=1  boolean_output=off  mode=Upper Bit Location + Width  bit1=3  base1=LSB of Input  bit0=0  base0=LSB of Input  XmcBlockStatus=1  maskContainerNames=group1  block_type=slice  block_config=sysgen:Slice_config
  Subsystem Reference{,1..3} (4 alike) : Subsystem  ReferencedSubsystem=ALU_1bit_SS
      settings: PortSchema="{\"entries\":[{\"content\":{\"sides\":[{\"content\":{\"connectorIds\":[\"In4\",\"In5\"]},\"type\":\"ConnectorPlacement.EquallySpacedRectSide\",\"uuid\":\"2d8c2f3b-1550-46fa-bff2-1c6af3b5a107\"},{\"content\":{\"connectorIds\":[\"Out1\",\"Out2\"],\"side\":\"RIGHT\"},\"type\":\"ConnectorPlacement.EquallySpacedRectSide\",\"uuid\":\"4b8f41aa-218a-4e29-bd3a-77a8547f4b37\"},{\"content\":{\"connectorIds\":[\"In1\",\"In3\",\"In2\",\"In6\"],\"side\":\"TOP\"},\"type\":\"ConnectorPlacement.EquallySpacedRectSide\",\"uuid\":\"e119eb8d-dd79-436a-880b-8e6ed91d7b6a\"}]},\"type\":\"ConnectorPlacement.EquallySpacedConnector\",\"uuid\":\"6756e4eb-c638-4708-925d-61f35342c635\"}],\"packageUris\":[\"http://schema.mathworks.com/mf0/Connector/R2020b\"],\"version\":\"1.0\"}"
  result : Outport
  CarryOut : Outport  Port=2
  wires:
  Subsystem Reference3/1 -> Concat/1
  Subsystem Reference1/1 -> Concat/3
  Op/1 -> Subsystem Reference1/1, Subsystem Reference2/1, Subsystem Reference3/1, Subsystem Reference/1
  a/1 -> Slice/1, Slice2/1, Slice4/1, Slice6/1
  CarryIn/1 -> Subsystem Reference/6
  Binv/1 -> Subsystem Reference1/3, Subsystem Reference2/3, Subsystem Reference3/3, Subsystem Reference/3
  Ainv/1 -> Subsystem Reference1/2, Subsystem Reference2/2, Subsystem Reference3/2, Subsystem Reference/2
  Concat/1 -> result/1
  Slice4/1 -> Subsystem Reference2/4
  Subsystem Reference2/1 -> Concat/2
  Subsystem Reference1/2 -> Subsystem Reference2/6
  Slice6/1 -> Subsystem Reference3/4
  Slice7/1 -> Subsystem Reference3/5
  Slice5/1 -> Subsystem Reference2/5
  b/1 -> Slice1/1, Slice3/1, Slice5/1, Slice7/1
  Subsystem Reference/2 -> Subsystem Reference1/6
  Subsystem Reference2/2 -> Subsystem Reference3/6
  Subsystem Reference/1 -> Concat/4
  Slice/1 -> Subsystem Reference/4
  Subsystem Reference3/2 -> CarryOut/1
  Slice3/1 -> Subsystem Reference1/5
  Slice1/1 -> Subsystem Reference/5
  Slice2/1 -> Subsystem Reference1/4

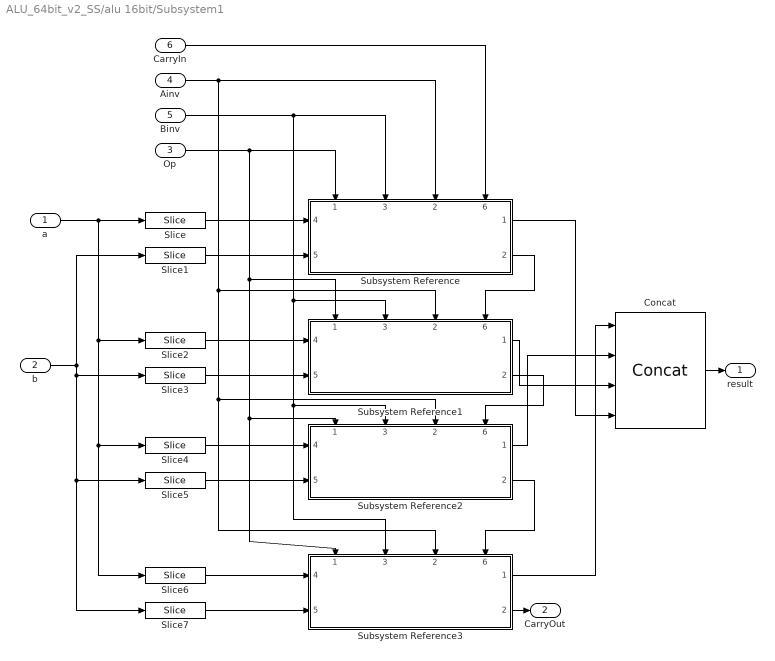
== system ALU_64bit_v2_SS/alu 16bit/Subsystem1 ==
  a : Inport
  b : Inport  Port=2
  Op : Inport  Port=3
  Ainv : Inport  Port=4
  Binv : Inport  Port=5
  CarryIn : Inport  Port=6
  Concat : hdlBasic/Concat  num_inputs=4  XmcBlockStatus=1  maskContainerNames=group1  block_type=concat  block_config=sysgen:Concat_config
  Slice : hdlBasic/Slice  nbits=1  boolean_output=off  mode=Upper Bit Location + Width  bit1=0  base1=LSB of Input  bit0=0  base0=LSB of Input  XmcBlockStatus=1  maskContainerNames=group1  block_type=slice  block_config=sysgen:Slice_config
  Slice1 : hdlBasic/Slice  nbits=1  boolean_output=off  mode=Upper Bit Location + Width  bit1=0  base1=LSB of Input  bit0=0  base0=LSB of Input  XmcBlockStatus=1  maskContainerNames=group1  block_type=slice  block_config=sysgen:Slice_config
  Slice2 : hdlBasic/Slice  nbits=1  boolean_output=off  mode=Upper Bit Location + Width  bit1=1  base1=LSB of Input  bit0=0  base0=LSB of Input  XmcBlockStatus=1  maskContainerNames=group1  block_type=slice  block_config=sysgen:Slice_config
  Slice3 : hdlBasic/Slice  nbits=1  boolean_output=off  mode=Upper Bit Location + Width  bit1=1  base1=LSB of Input  bit0=0  base0=LSB of Input  XmcBlockStatus=1  maskContainerNames=group1  block_type=slice  block_config=sysgen:Slice_config
  Slice4 : hdlBasic/Slice  nbits=1  boolean_output=off  mode=Upper Bit Location + Width  bit1=2  base1=LSB of Input  bit0=0  base0=LSB of Input  XmcBlockStatus=1  maskContainerNames=group1  block_type=slice  block_config=sysgen:Slice_config
  Slice5 : hdlBasic/Slice  nbits=1  boolean_output=off  mode=Upper Bit Location + Width  bit1=2  base1=LSB of Input  bit0=0  base0=LSB of Input  XmcBlockStatus=1  maskContainerNames=group1  block_type=slice  block_config=sysgen:Slice_config
  Slice6 : hdlBasic/Slice  nbits=1  boolean_output=off  mode=Upper Bit Location + Width  bit1=3  base1=LSB of Input  bit0=0  base0=LSB of Input  XmcBlockStatus=1  maskContainerNames=group1  block_type=slice  block_config=sysgen:Slice_config
  Slice7 : hdlBasic/Slice  nbits=1  boolean_output=off  mode=Upper Bit Location + Width  bit1=3  base1=LSB of Input  bit0=0  base0=LSB of Input  XmcBlockStatus=1  maskContainerNames=group1  block_type=slice  block_config=sysgen:Slice_config
  Subsystem Reference{,1..3} (4 alike) : Subsystem  ReferencedSubsystem=ALU_1bit_SS
      settings: PortSchema="{\"entries\":[{\"content\":{\"sides\":[{\"content\":{\"connectorIds\":[\"In4\",\"In5\"]},\"type\":\"ConnectorPlacement.EquallySpacedRectSide\",\"uuid\":\"2d8c2f3b-1550-46fa-bff2-1c6af3b5a107\"},{\"content\":{\"connectorIds\":[\"Out1\",\"Out2\"],\"side\":\"RIGHT\"},\"type\":\"ConnectorPlacement.EquallySpacedRectSide\",\"uuid\":\"4b8f41aa-218a-4e29-bd3a-77a8547f4b37\"},{\"content\":{\"connectorIds\":[\"In1\",\"In3\",\"In2\",\"In6\"],\"side\":\"TOP\"},\"type\":\"ConnectorPlacement.EquallySpacedRectSide\",\"uuid\":\"e119eb8d-dd79-436a-880b-8e6ed91d7b6a\"}]},\"type\":\"ConnectorPlacement.EquallySpacedConnector\",\"uuid\":\"6756e4eb-c638-4708-925d-61f35342c635\"}],\"packageUris\":[\"http://schema.mathworks.com/mf0/Connector/R2020b\"],\"version\":\"1.0\"}"
  result : Outport
  CarryOut : Outport  Port=2
  wires:
  Subsystem Reference3/1 -> Concat/1
  Subsystem Reference1/1 -> Concat/3
  Op/1 -> Subsystem Reference1/1, Subsystem Reference2/1, Subsystem Reference3/1, Subsystem Reference/1
  a/1 -> Slice/1, Slice2/1, Slice4/1, Slice6/1
  CarryIn/1 -> Subsystem Reference/6
  Binv/1 -> Subsystem Reference1/3, Subsystem Reference2/3, Subsystem Reference3/3, Subsystem Reference/3
  Ainv/1 -> Subsystem Reference1/2, Subsystem Reference2/2, Subsystem Reference3/2, Subsystem Reference/2
  Concat/1 -> result/1
  Slice4/1 -> Subsystem Reference2/4
  Subsystem Reference2/1 -> Concat/2
  Subsystem Reference1/2 -> Subsystem Reference2/6
  Slice6/1 -> Subsystem Reference3/4
  Slice7/1 -> Subsystem Reference3/5
  Slice5/1 -> Subsystem Reference2/5
  b/1 -> Slice1/1, Slice3/1, Slice5/1, Slice7/1
  Subsystem Reference/2 -> Subsystem Reference1/6
  Subsystem Reference2/2 -> Subsystem Reference3/6
  Subsystem Reference/1 -> Concat/4
  Slice/1 -> Subsystem Reference/4
  Subsystem Reference3/2 -> CarryOut/1
  Slice3/1 -> Subsystem Reference1/5
  Slice1/1 -> Subsystem Reference/5
  Slice2/1 -> Subsystem Reference1/4

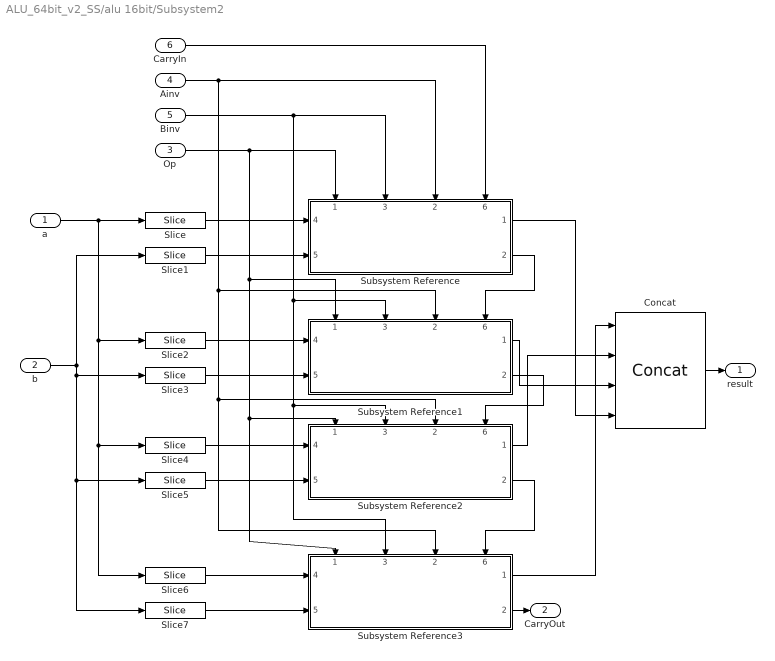
== system ALU_64bit_v2_SS/alu 16bit/Subsystem2 ==
  a : Inport
  b : Inport  Port=2
  Op : Inport  Port=3
  Ainv : Inport  Port=4
  Binv : Inport  Port=5
  CarryIn : Inport  Port=6
  Concat : hdlBasic/Concat  num_inputs=4  XmcBlockStatus=1  maskContainerNames=group1  block_type=concat  block_config=sysgen:Concat_config
  Slice : hdlBasic/Slice  nbits=1  boolean_output=off  mode=Upper Bit Location + Width  bit1=0  base1=LSB of Input  bit0=0  base0=LSB of Input  XmcBlockStatus=1  maskContainerNames=group1  block_type=slice  block_config=sysgen:Slice_config
  Slice1 : hdlBasic/Slice  nbits=1  boolean_output=off  mode=Upper Bit Location + Width  bit1=0  base1=LSB of Input  bit0=0  base0=LSB of Input  XmcBlockStatus=1  maskContainerNames=group1  block_type=slice  block_config=sysgen:Slice_config
  Slice2 : hdlBasic/Slice  nbits=1  boolean_output=off  mode=Upper Bit Location + Width  bit1=1  base1=LSB of Input  bit0=0  base0=LSB of Input  XmcBlockStatus=1  maskContainerNames=group1  block_type=slice  block_config=sysgen:Slice_config
  Slice3 : hdlBasic/Slice  nbits=1  boolean_output=off  mode=Upper Bit Location + Width  bit1=1  base1=LSB of Input  bit0=0  base0=LSB of Input  XmcBlockStatus=1  maskContainerNames=group1  block_type=slice  block_config=sysgen:Slice_config
  Slice4 : hdlBasic/Slice  nbits=1  boolean_output=off  mode=Upper Bit Location + Width  bit1=2  base1=LSB of Input  bit0=0  base0=LSB of Input  XmcBlockStatus=1  maskContainerNames=group1  block_type=slice  block_config=sysgen:Slice_config
  Slice5 : hdlBasic/Slice  nbits=1  boolean_output=off  mode=Upper Bit Location + Width  bit1=2  base1=LSB of Input  bit0=0  base0=LSB of Input  XmcBlockStatus=1  maskContainerNames=group1  block_type=slice  block_config=sysgen:Slice_config
  Slice6 : hdlBasic/Slice  nbits=1  boolean_output=off  mode=Upper Bit Location + Width  bit1=3  base1=LSB of Input  bit0=0  base0=LSB of Input  XmcBlockStatus=1  maskContainerNames=group1  block_type=slice  block_config=sysgen:Slice_config
  Slice7 : hdlBasic/Slice  nbits=1  boolean_output=off  mode=Upper Bit Location + Width  bit1=3  base1=LSB of Input  bit0=0  base0=LSB of Input  XmcBlockStatus=1  maskContainerNames=group1  block_type=slice  block_config=sysgen:Slice_config
  Subsystem Reference{,1..3} (4 alike) : Subsystem  ReferencedSubsystem=ALU_1bit_SS
      settings: PortSchema="{\"entries\":[{\"content\":{\"sides\":[{\"content\":{\"connectorIds\":[\"In4\",\"In5\"]},\"type\":\"ConnectorPlacement.EquallySpacedRectSide\",\"uuid\":\"2d8c2f3b-1550-46fa-bff2-1c6af3b5a107\"},{\"content\":{\"connectorIds\":[\"Out1\",\"Out2\"],\"side\":\"RIGHT\"},\"type\":\"ConnectorPlacement.EquallySpacedRectSide\",\"uuid\":\"4b8f41aa-218a-4e29-bd3a-77a8547f4b37\"},{\"content\":{\"connectorIds\":[\"In1\",\"In3\",\"In2\",\"In6\"],\"side\":\"TOP\"},\"type\":\"ConnectorPlacement.EquallySpacedRectSide\",\"uuid\":\"e119eb8d-dd79-436a-880b-8e6ed91d7b6a\"}]},\"type\":\"ConnectorPlacement.EquallySpacedConnector\",\"uuid\":\"6756e4eb-c638-4708-925d-61f35342c635\"}],\"packageUris\":[\"http://schema.mathworks.com/mf0/Connector/R2020b\"],\"version\":\"1.0\"}"
  result : Outport
  CarryOut : Outport  Port=2
  wires:
  Subsystem Reference3/1 -> Concat/1
  Subsystem Reference1/1 -> Concat/3
  Op/1 -> Subsystem Reference1/1, Subsystem Reference2/1, Subsystem Reference3/1, Subsystem Reference/1
  a/1 -> Slice/1, Slice2/1, Slice4/1, Slice6/1
  CarryIn/1 -> Subsystem Reference/6
  Binv/1 -> Subsystem Reference1/3, Subsystem Reference2/3, Subsystem Reference3/3, Subsystem Reference/3
  Ainv/1 -> Subsystem Reference1/2, Subsystem Reference2/2, Subsystem Reference3/2, Subsystem Reference/2
  Concat/1 -> result/1
  Slice4/1 -> Subsystem Reference2/4
  Subsystem Reference2/1 -> Concat/2
  Subsystem Reference1/2 -> Subsystem Reference2/6
  Slice6/1 -> Subsystem Reference3/4
  Slice7/1 -> Subsystem Reference3/5
  Slice5/1 -> Subsystem Reference2/5
  b/1 -> Slice1/1, Slice3/1, Slice5/1, Slice7/1
  Subsystem Reference/2 -> Subsystem Reference1/6
  Subsystem Reference2/2 -> Subsystem Reference3/6
  Subsystem Reference/1 -> Concat/4
  Slice/1 -> Subsystem Reference/4
  Subsystem Reference3/2 -> CarryOut/1
  Slice3/1 -> Subsystem Reference1/5
  Slice1/1 -> Subsystem Reference/5
  Slice2/1 -> Subsystem Reference1/4
